simulink model "Loop_detailed_model_comp_cc_vccc_v13"  (R2013a)
settings: Solver=ode23  SolverMode=SingleTasking  StartTime=0.0  StopTime=8e-3  FixedStep=FS/250  MaxStep=1e-4  RelTol=1e-3
InitFcn:
  | %%%%%%  set scope time range
  | T_STOP=str2num(get_param(gcs,'StopTime'));
  | if numel(T_STOP) > 1
  |    T_STOP=T_STOP(2);
  | else
  |    T_STOP=T_STOP(1);
  | end
  | T_STOP=num2str(T_STOP);
  | 
  | %%%%%%  set scope time range in system @init_callback_fct
  | T_STOP=num2str(str2num(get_param(gcs,'StopTime')));
  | 
  | childs = allchild(0);
  | sol=strfind(upper(get(allchild(0),'Tag')),'VIEWER_PARAMETERS');
  | 
  | if iscell(sol)
  |    ind=find(~cellfun(@isempty, strfind(upper(get(allchild(0),'Tag')),'VIEWER_PARAMETERS')));
  | else
  |    ind=sol;
  | end
  | %ind=find(~cellfun(@isempty, {strfind(upper(get(allchild(0),'Tag')),'VIEWER_PARAMETERS'),[]}))
  | if ~isempty(ind)
  |    for k=1:length(childs(ind))
  |       set_param(getfield(get(childs(ind(k)),'UserData'),'block'),'TimeRange', T_STOP);
  | %      get_param(getfield(get(childs(ind(k)),'UserData'),'block'),'TimeRange');
  | %    set_param(getfield(get(childs(ind),'UserData'),'block'),'TimeRange',T_STOP);
  | %    get_param(getfield(get(childs(ind),'UserData'),'block'),'TimeRange');
  |    end
  | else
  |     warning(sprintf('VIEWER_PARAMETERS object not found\nOpen the config dialog by hand for the first sim start'))
  | end
values from neighbouring files (symbols this model uses):
  FS = 5e-6    (= 5e-06)    [GalvoModel_v4_sys.m]    (also in GalvoModel_v6_sys.m = 5e-05; Galvo_process_analyze.m = 0.0001)
  Lc = 170e-6    (= 0.00017)    [GalvoModel_v6_sys.m]    (also in Galvo_process_analyze.m)
  Rc = 1.5    [GalvoModel_v6_sys.m]    (also in Galvo_process_analyze.m; frequenzgang_nichtinvert_opamp_koblitz_eas.m = 1)
  Rsh = 0.003    [GalvoModel_v6_sys.m]    (also in Galvo_sys_proto_v13_OFFSETS_MODEL_PT1B_proc.m = 0.075; frequenzgang_nichtinvert_opamp_koblitz_eas.m = 0.015)
libraries: simulink x2
settings Model: BufferReuse=off  Creator=mainster  LastModifiedBy=mainster
settings SolverCC: AutoInsertRateTranBlk=on
settings OptimizationCC: InlineParams=on  BufferReuse=off
settings DebuggingCC: InitInArrayFormatMsg=none
settings HardwareCC: ProdLargestAtomicInteger=Long  ProdLargestAtomicFloat=Double  ProdEndianess=LittleEndian  ProdHWDeviceType=ARM Compatible->ARM Cortex

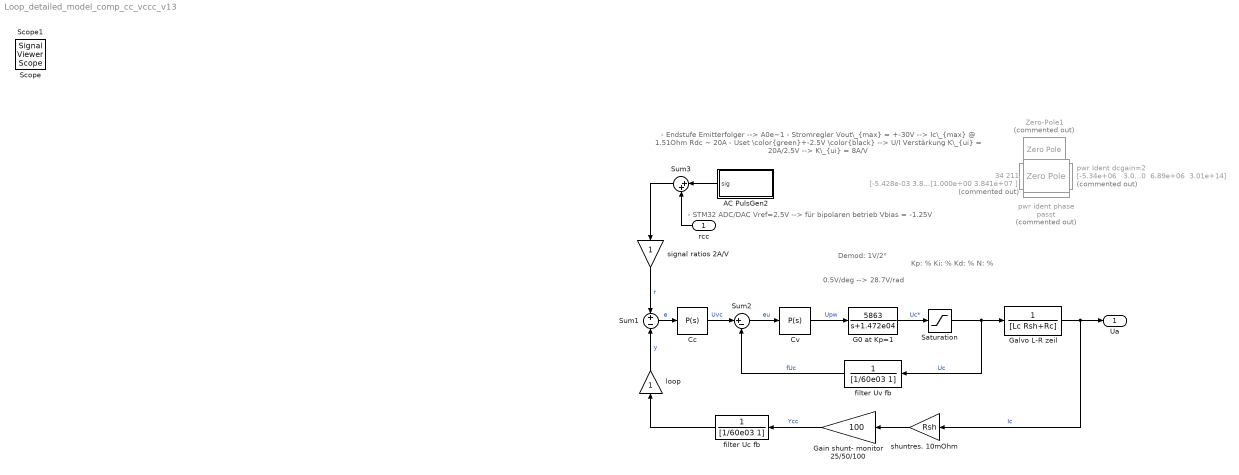
== system Loop_detailed_model_comp_cc_vccc_v13 ==
  note: - Endstufe Emitterfolger --> A0e~1
      | - Stromregler Vout\_{max} = +-30V
      |       --> Ic\_{max} @ 1.51Ohm Rdc ~ 20A
      | - Uset \color{green}+-2.5V \color{black}
      |       --> U/I Verstärkung K\_{ui} = 20A/2.5V
      |       --> K\_{ui} = 8A/V
  note: - STM32 ADC/DAC Vref=2.5V
      | --> für bipolaren betrieb Vbias = -1.25V
  note: Kp: % Ki: % Kd: % N: %
  note: 0.5V/deg --> 28.7V/rad
  note: Demod:
      | 1V/2°
  rcc : Inport
  34 211 : TransferFcn  Commented=on  Numerator=[-5.428e-03 3.828e+07 ]/[-5.428e-03 3.828e+07 ]  Denominator=[1.000e+00 3.841e+07 ]/[1.000e+00 3.841e+07 ]
  AC PulsGen2 : Subsystem  mask{sigp=10, sigpp=0, offs=0}
      mask prompts: sigp "Insert signal peak"; sigpp "or signal peak-to-peak"; offs "Insert DC offset"
      mask TypeOptions sigp: PulsGen/Amplitude
      mask Callback sigp:
      | %sigp=get_param([gcb '/PulsGen'],'Amplitude')
      | %SigVal=2*sigp
      mask TypeOptions offs: offset/Value
      mask Display:
      | %str=sprintf('%s',get(gcbh,'ModelName'));
      | port_label('output', 1, '','texmode','off')
      | %text(.05,.98,['{\fontsize{12}\it\bf' strrep(str,'_',' ') '}'],'horizontalAlignment','left','verticalAlignment','top','texmode','on')
      | %text(.5,0.95,['{\fontsize{8}A_{peak}=}'],'horizontalAlignment','center','verticalAlignment','top','texmode','on')
      | disp(sprintf('Up=%.3g\nDC=%.3g',sigp, offs))
      | %disp(['Upp=' sigpp])%, offs))
      | %sprintf('sigpp==%s',sigpp)
      | %text(.15,.05,['{\fontsize{10}\itmechanics}'],'horizontalAlignment','left','verticalAlignment','bottom','texmode','on')
  Cc : simulink/Continuous/PID Controller  Controller=P  TimeDomain=Continuous-time  SampleTime=1  IntegratorMethod=Forward Euler  FilterMethod=Forward Euler  Form=Parallel  P=7.60182030835902  I=1  D=0  N=100  InitialConditionSource=internal  InitialConditionForIntegrator=0  InitialConditionForFilter=0  ExternalReset=none  LimitOutput=on  UpperSaturationLimit=30  LowerSaturationLimit=-30  LinearizeAsGain=on  AntiWindupMode=none  Kb=1  TrackingMode=off  Kt=1  PParamMin=[]  PParamMax=[]  IParamMin=[]  IParamMax=[]  DParamMin=[]  DParamMax=[]  NParamMin=[]  NParamMax=[]  KbParamMin=[]  KbParamMax=[]  KtParamMin=[]  KtParamMax=[]  POutMin=[]  POutMax=[]  IOutMin=[]  IOutMax=[]  DOutMin=[]  DOutMax=[]  NOutMin=[]  NOutMax=[]  KbOutMin=[]  KbOutMax=[]  KtOutMin=[]  KtOutMax=[]  IntegratorOutMin=[]  IntegratorOutMax=[]  FilterOutMin=[]  FilterOutMax=[]  SumOutMin=[]  SumOutMax=[]  SumI1OutMin=[]  SumI1OutMax=[]  SumI2OutMin=[]  SumI2OutMax=[]  SumI3OutMin=[]  SumI3OutMax=[]  SumDOutMin=[]  SumDOutMax=[]  SaturationOutMin=[]  SaturationOutMax=[]  IntegratorContinuousStateAttributes=''  IntegratorStateMustResolveToSignalObject=off  IntegratorRTWStateStorageClass=Auto  FilterContinuousStateAttributes=''  FilterStateMustResolveToSignalObject=off  FilterRTWStateStorageClass=Auto
  Cv : simulink/Continuous/PID Controller  Controller=P  TimeDomain=Continuous-time  SampleTime=1  IntegratorMethod=Forward Euler  FilterMethod=Forward Euler  Form=Parallel  P=14.3035575429842  I=1  D=0  N=100  InitialConditionSource=internal  InitialConditionForIntegrator=0  InitialConditionForFilter=0  ExternalReset=none  LimitOutput=on  UpperSaturationLimit=30  LowerSaturationLimit=-30  LinearizeAsGain=on  AntiWindupMode=none  Kb=1  TrackingMode=off  Kt=1  PParamMin=[]  PParamMax=[]  IParamMin=[]  IParamMax=[]  DParamMin=[]  DParamMax=[]  NParamMin=[]  NParamMax=[]  KbParamMin=[]  KbParamMax=[]  KtParamMin=[]  KtParamMax=[]  POutMin=[]  POutMax=[]  IOutMin=[]  IOutMax=[]  DOutMin=[]  DOutMax=[]  NOutMin=[]  NOutMax=[]  KbOutMin=[]  KbOutMax=[]  KtOutMin=[]  KtOutMax=[]  IntegratorOutMin=[]  IntegratorOutMax=[]  FilterOutMin=[]  FilterOutMax=[]  SumOutMin=[]  SumOutMax=[]  SumI1OutMin=[]  SumI1OutMax=[]  SumI2OutMin=[]  SumI2OutMax=[]  SumI3OutMin=[]  SumI3OutMax=[]  SumDOutMin=[]  SumDOutMax=[]  SaturationOutMin=[]  SaturationOutMax=[]  IntegratorContinuousStateAttributes=''  IntegratorStateMustResolveToSignalObject=off  IntegratorRTWStateStorageClass=Auto  FilterContinuousStateAttributes=''  FilterStateMustResolveToSignalObject=off  FilterRTWStateStorageClass=Auto
  G0 at Kp=1 : TransferFcn  Numerator=5863  Denominator="[1  1.472e04]"
  Gain shunt- monitor 25/50/100 : Gain  Gain=100  SampleTime=0
  Galvo L-R zeil : TransferFcn  Numerator=1  Denominator=[Lc Rsh+Rc]
  Saturation : Saturate  UpperLimit=35  LowerLimit=-35
  Sum1 : Sum  Inputs=+|-  SampleTime=0
  Sum2 : Sum  Inputs=|+-
  Sum3 : Sum  Inputs=|++  SampleTime=0
  Zero-Pole1 : ZeroPole  Commented=on  Zeros=-5.618e7  Poles=[-0.3445+1.7004i -0.3445-1.7004i]
  filter Uc fb : TransferFcn  Denominator=[1/60e03 1]
  filter Uv fb : TransferFcn  Denominator=[1/60e03 1]
  loop : Gain  SampleTime=0
  pwr Ident dcgain=2 : TransferFcn  Commented=on  Numerator="[-5.34e+06   3.00e+14]"  Denominator="[1.00e+00  6.89e+06  3.01e+14]"
  pwr ident phase passt : ZeroPole  Commented=on  Zeros=[]  Poles=[-7.2010 -0.0385]*1e9  Gain=2.76e17
  shuntres. 10mOhm : Gain  Gain=Rsh  SampleTime=0
  signal ratios 2A/V : Gain  SampleTime=0
  Ua : Outport  SampleTime=0
  Scope : SignalViewerScope  IOType=viewer  NumInputPorts=4  LegendLocations=|  RefreshTime=0.035000
      | 0.70754     0.93444     0.10921    0.038639
      | 0.81715     0.69875     0.13087    0.038639
      | 0.81715     0.46306     0.13087    0.021692
      | 0.82717     0.22804     0.12004    0.021692
      settings: ShowLegends=on  TimeRange=0.008  YMin=-10~-1.5~-2~-1  YMax=10~1.5~2~1
  Scope1 : SignalViewerScope  IOType=viewer  NumInputPorts=2  LegendLocations="0.80057     0.89997     0.19444    0.048662 0.80057     0.43879     0.19444    0.048662"  RefreshTime=0.035000
      settings: ShowLegends=on  TimeRange=0.008  YMin=-5~-5  YMax=5~5
  wires:
  Galvo L-R zeil/1 -> shuntres. 10mOhm/1, Ua/1  "Ic"
  Cv/1 -> G0 at Kp=1/1  "Upw"
  G0 at Kp=1/1 -> Saturation/1  "Uc*"
  Sum1/1 -> Cc/1  "e"
  Gain shunt- monitor 25/50/100/1 -> filter Uc fb/1  "Ycc"
  shuntres. 10mOhm/1 -> Gain shunt- monitor 25/50/100/1
  signal ratios 2A/V/1 -> Sum1/1  "r"
  Sum2/1 -> Cv/1  "eu"
  Cc/1 -> Sum2/1  "Uvc"
  filter Uv fb/1 -> Sum2/2  "fUc"
  AC PulsGen2/1(sig) -> Sum3/1
  Sum3/1 -> signal ratios 2A/V/1
  rcc/1 -> Sum3/2
  loop/1 -> Sum1/2  "y"
  Saturation/1 -> Galvo L-R zeil/1, filter Uv fb/1  "Uc"
  filter Uc fb/1 -> loop/1

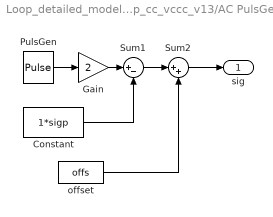
== system Loop_detailed_model_comp_cc_vccc_v13/AC PulsGen2 ==
  Constant : Constant  Value=1*sigp
  Gain : Gain  Gain=2
  PulsGen : DiscretePulseGenerator  PulseType=Time based  Amplitude=sigp  Period=4e-3  PulseWidth=50  PhaseDelay=0.5e-3  SampleTime=FS
      settings: AttributesFormatString=A=%<Amplitude>\nPeri=%<Period>
  Sum1 : Sum  Inputs=|+-
  Sum2 : Sum  Inputs=|++
  offset : Constant  Value=offs
  sig : Outport
  wires:
  Sum2/1 -> sig/1
  PulsGen/1 -> Gain/1
  offset/1 -> Sum2/2
  Gain/1 -> Sum1/1
  Sum1/1 -> Sum2/1
  Constant/1 -> Sum1/2
